simulink model "S2_Boost_model_real"  (R2021a)
settings: Solver=VariableStepAuto  StartTime=0.0  StopTime=spec.sim_time  FixedStep=1e-9  MaxStep=1e-7  RelTol=1e-3
undefined symbols (not defined in the file): real, spec
libraries: fl_lib x16, nesl_utility x12, spsMeanLib x5, ee_lib x4, spsRMSLib x3, spsPWMGeneratorDCDCLib x1
settings Model: Creator=delta  LastModifiedBy=delta
settings SolverCC: MaxConsecutiveMinStep=10  ZeroCrossAlgorithm=Adaptive
settings DebuggingCC: IgnoredZcDiagnostic=none

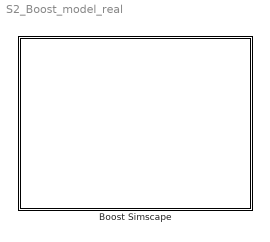
== system S2_Boost_model_real ==
  Boost Simscape : Subsystem

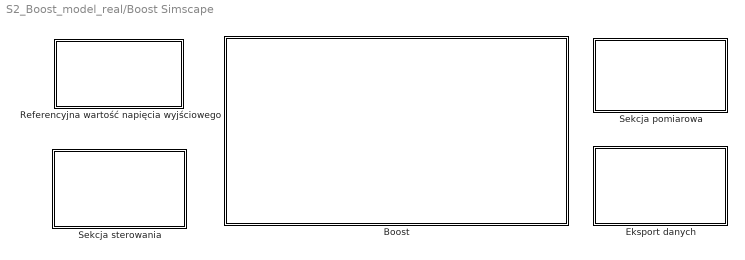
== system S2_Boost_model_real/Boost Simscape ==
  Boost : Subsystem
  Eksport danych : Subsystem
  Referencyjna wartość napięcia wyjściowego : Subsystem
  Sekcja pomiarowa : Subsystem
  Sekcja sterowania : Subsystem

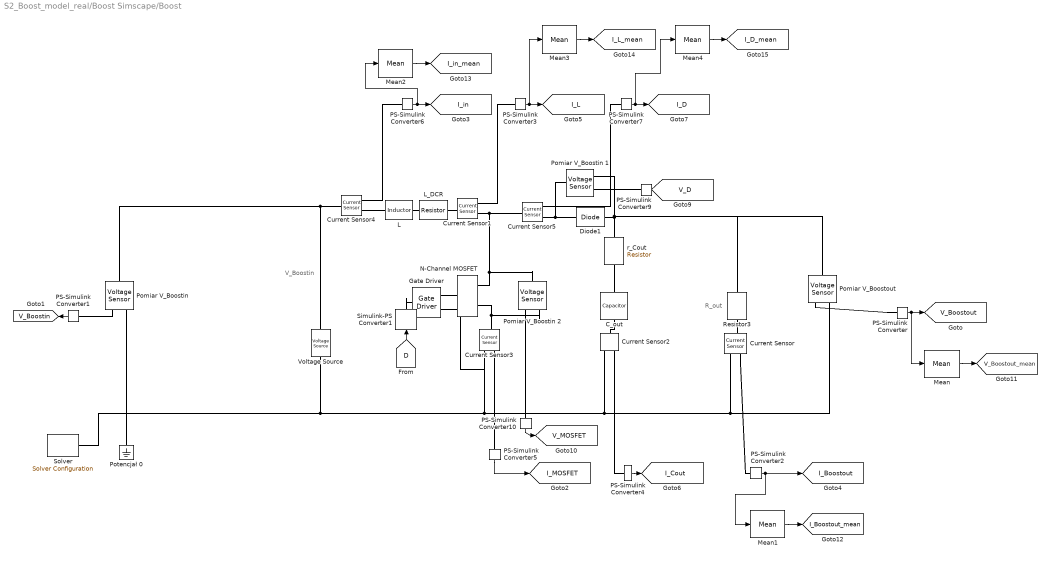
== system S2_Boost_model_real/Boost Simscape/Boost ==
  note: V_Boostin
  note: R_out
  "C_out " : fl_lib/Electrical/Electrical Elements/Capacitor  c=real.Cout.param.C_out F  r=0 Ohm  g=0 1/Ohm  i_specify=off  i_priority=None  i=0 A  i_nominal_specify=off  i_nominal_unit=A  i_nominal_value=1  v_specify=off  v_priority=None  v=0 V  v_nominal_specify=off  v_nominal_unit=V  v_nominal_value=1  vc_specify=off  vc_priority=High  vc=0 V  vc_nominal_specify=off  vc_nominal_unit=V  vc_nominal_value=1
  Current Sensor{,1..5} (6 alike) : fl_lib/Electrical/Electrical Sensors/Current Sensor
  Diode1 : ee_lib/Semiconductors & Converters/Diode  ModelType=ee.enum.diode.modelType.pwl  IfMat=[.07, .12, .19, 1.75, 4.24, 7.32, 11.2; .16, .3, .72, 2.14, 4.02, 6.35, 9.12] A  TjVec=[25, 125] degC  VfVec=[.5, .7, .9, 1.3, 1.7, 2.1, 2.5] V  Vf=real.Diode.param.V_f V  Ron=1e-9 Ohm  Goff=1e-8 S  prmExp=ee.enum.diode.expParam.useTwo  I12=[.0137, .545] A  V12=[.6, .7] V  IS=1e-12 A  ec=1  I1=0.0137 A  V1=0.6 V  RS=0 Ohm  Tmeas=25 degC  N_series=1  N_parallel=1  Rz=0.3 Ohm  BV=inf V  C_param=ee.enum.diode.capParam.fixed  CJ=5 pF  CJ0=5 pF  VJ=1 V  Mgrad=0.5  Vvec=[.1, 10, 100] V  Cvec=[3.5, 1, .4] pF  FC=0.5  Q_param=ee.enum.diode.recoveryParam.off  iRM=-7.15 A  iF=4 A  didt=-750 A/us  trr_factor=3  trr=115 ns  Qrr=150 s*nA  TT=50 ns  tau=100 ns  T_param=ee.enum.diode.temperatureParam.off  IS_T2=1.25e-7 A  I1_T2=0.245 A  V1_T2=0.5 V  Tmeas2=125 degC  EG_param=ee.enum.diode.egapParam.material_si  EG=1.11 eV  XTI_param=ee.enum.diode.xtiParam.pn  XTI=3  dBVdT=0 V/K  enable_faults=ee.enum.faults.faultEnable.no  fault_action=ee.enum.faults.faultAction.none  fault_types=ee.enum.diode.faults.open  tau_fault=1e-3 s  IfMat_faulted=[.07, .12, .19, 1.75, 4.24, 7.32, 11.2; .16, .3, .72, 2.14, 4.02, 6.35, 9.12] A  VfVec_faulted=[.5, .7, .9, 1.3, 1.7, 2.1, 2.5] V  Ropen_faulted=1000 Ohm  Gshort_faulted=1000 1/Ohm  Vf_faulted=0.6 V  Ron_faulted=0.3 Ohm  Goff_faulted=1e-8 S  I12_faulted=[.0137, .545] A  V12_faulted=[.6, .7] V  IS_faulted=1e-12 A  ec_faulted=1  I1_faulted=0.0137 A  V1_faulted=0.6 V  RS_faulted=0 Ohm  Rz_faulted=0.3 Ohm  BV_faulted=inf V  Cscale_faulted=100  enable_temporal_fault=ee.enum.faults.faultEnable.no  t_fault=inf s  enable_behavioral_fault=ee.enum.faults.faultEnable.no  max_permissible_voltage=inf V  n_fail_on_voltage=1  max_permissible_current=inf A  t_fail_on_current=1 s  max_permissible_dVdt=inf V/s  Tdevice=25 degC  i_specify=off  i_priority=None  i=0 A  i_nominal_specify=off  i_nominal_unit=A  i_nominal_value=1  v_specify=off  v_priority=None  v=0 V  v_nominal_specify=off  v_nominal_unit=V  v_nominal_value=1  i_diode_specify=off  i_diode_priority=None  i_diode=0 A  i_diode_nominal_specify=off  i_diode_nominal_unit=A  i_diode_nominal_value=1  v_diode_specify=off  v_diode_priority=None  v_diode=0 V  v_diode_nominal_specify=off  v_diode_nominal_unit=V  v_diode_nominal_value=1  i_capacitor_specify=off  i_capacitor_priority=None  i_capacitor=0 A  i_capacitor_nominal_specify=off  i_capacitor_nominal_unit=A  i_capacitor_nominal_value=1  v_capacitor_specify=off  v_capacitor_priority=None  v_capacitor=0 V  v_capacitor_nominal_specify=off  v_capacitor_nominal_unit=V  v_capacitor_nominal_value=1  power_dissipated_specify=off  power_dissipated_priority=None  power_dissipated=0 W  power_dissipated_nominal_specify=off  power_dissipated_nominal_unit=W  power_dissipated_nominal_value=1  max_permissible_temperature=inf K  t_fail_on_temperature=1 s  thermal_network_parameterization=ee.enum.thermalNetworkTopology.cauer  Rth=[0, 10] K/W  Rth_Foster=[4, 6] K/W  thermal_mass_parameterization=ee.enum.thermalNetwork.timeconstant  thermal_mass=[0, 1] J/K  thermal_mass_Foster=[1.5, 3] J/K  thermal_time_constant=[0, 10] s  thermal_time_constant_Foster=[6, 18] s  thermal_mass_initial_temperatures=[25, 25] degC
  Gate Driver : ee_lib/Semiconductors & Converters/Gate Driver  vHigh=real.MOSFET.param.V_GS V  vLow=0 V  parameterization=2  rHigh=1e-9 Ohm  rLow=1e-9 Ohm  tRise=real.MOSFET.param.t_R s  tFall=real.MOSFET.param.t_F s  cLoad=10 nF  enable_faults=0  t_fault=1 s  fault_type=1  uHighValue=0.7  uLowValue=0.3  tHigh=real.MOSFET.param.t_R s  tLow=real.MOSFET.param.t_F s  ZonTime_specify=off  ZonTime_priority=None  ZonTime=0 s  ZoffTime_specify=off  ZoffTime_priority=None  ZoffTime=0 s  uHigh=2.0 V  uLow=0.8 V
      settings: SourceProductBaseCode=PS  InternalSimscapePortConfiguration="{\"Bottom\":[],\"Left\":[{\"id\":\"u\",\"label\":\"u\",\"type\":\"input\"}],\"Right\":[{\"id\":\"G\",\"label\":\"G\",\"type\":\"foundation.electrical.electrical\"},{\"id\":\"S\",\"label\":\"S\",\"type\":\"foundation.electrical.electrical\"}],\"Top\":[]}"
  L : fl_lib/Electrical/Electrical Elements/Inductor  l=real.L.param.L H  r=0 Ohm  g=0 1/Ohm  i_specify=off  i_priority=None  i=0 A  i_nominal_specify=off  i_nominal_unit=A  i_nominal_value=1  v_specify=off  v_priority=None  v=0 V  v_nominal_specify=off  v_nominal_unit=V  v_nominal_value=1  i_L_specify=off  i_L_priority=High  i_L=0 A  i_L_nominal_specify=off  i_L_nominal_unit=A  i_L_nominal_value=1
  L_DCR : fl_lib/Electrical/Electrical Elements/Resistor  R=real.L.param.DCR Ohm  i_specify=off  i_priority=None  i=0 A  i_nominal_specify=off  i_nominal_unit=A  i_nominal_value=1  v_specify=off  v_priority=None  v=0 V  v_nominal_specify=off  v_nominal_unit=V  v_nominal_value=1
  Mean{,1..4} (5 alike) : spsMeanLib/Mean  Freq=spec.f_s  Vinit=0  Ts=0
  N-Channel MOSFET : ee_lib/Semiconductors & Converters/N-Channel MOSFET  paramTerminal=ee.enum.mosfet.numberOfTerminals.three  parameterization=ee.enum.mosfet.parameterization.datasheet  prmDatasheet=ee.enum.temperatureParameterization.none  prmEquCoeff=ee.enum.temperatureParameterization.none  Beta=5.0 A/V^2  Rds=real.MOSFET.param.R_DS Ohm  Id=real.MOSFET.param.I_D A  Vgs=real.MOSFET.param.V_GS V  Vth=real.MOSFET.param.V_th V  Vth0=1.7 V  lam=0 1/V  gamma_vth=0.5 V^0.50000  phib=0.5 V  Vth1=1.9071 V  Vbs1=-1 V  Vth2=2.066 V  Vbs2=-2 V  Tmeas=25 degC  RS=1e-9 Ohm  RD=1e-9 Ohm  RB=0.001 Ohm  C_param=ee.enum.mosfet.capacitanceParam.fixedciss  C_GS=270 pF  C_GD=80 pF  C_DS=0 pF  C_iss=real.MOSFET.param.C_iss F  C_rss=real.MOSFET.param.C_rss F  C_oss=real.MOSFET.param.C_oss F  charge_linearity_param=ee.enum.mosfet.cgdLinearity.constant  C_OX=200 pF  V_C_OX=-0.5 V  C_iss_vec=[720, 700, 590, 470, 390, 310] pF  C_rss_vec=[450, 400, 300, 190, 95, 55] pF  C_oss_vec=[900, 810, 690, 420, 270, 170] pF  C_GS_vec=[270, 300, 290, 280, 295, 255] pF  C_GD_vec=[450, 400, 300, 190, 95, 55] pF  C_DS_vec=[450, 410, 390, 230, 175, 115] pF  C_Vds_vec=[.1, .3, 1, 3, 10, 30] V  V_GS_for_cap_data=0 V  charge_linearity_param_vgb=ee.enum.mosfet.cgbLinearity.instantly  Di_param=ee.enum.mosfet.diodeParam.no  IsDiode=0 A  Vbi=0.6 V  n=1  Cj0Diode=0 pF  TT=50e-9 s  dVth_dT=-6 mV/K  dVth0_dT=-6 mV/K  Rds_T2=0.037 Ohm  Tmeas2=125 degC  BEXDatasheet=-1.5  BEXEquCoeff=-1.5  etaisDatasheet=3  etaisEquCoeff=3  Vgs_vec=[-.5, 2, 3, 4, 5] V  Vds_vec=[0, 2, 4, 8, 12, 16, 20] V  Vbs_vec=[0, -4, -6, -12] V  T_vec=[25, 125] degC  Vth_vec=[.4, 1.2, 1.4, 1.45] V  Vth_mat=[.4, .35; 1.2, 1.15; 1.4, 1.35; 1.45, 1.4] V  Ids_mat=[0, 0, 0, 0, 0, 0, 0; 0, .003, .0038, .0043, .0046, .0048, .0049; 0, .0055, .008, .009, .0095, .01, .0101; 0, .0115, .016, .018, .019, .0195, .02; 0, .0152, .0225, .0265, .028, .0295, .03] A  Ids_mat0=[0, 0, 0, 0, 0, 0, 0; 0, .003, .0038, .0043, .0046, .0048, .0049; 0, .0055, .008, .009, .0095, .01, .0101; 0, .0115, .016, .018, .019, .0195, .02; 0, .0152, .0225, .0265, .028, .0295, .03] A  Ids_mat_3D=zeros(5, 7, 2) A  Ids_mat_3D0=zeros(5, 7, 2) A  IV_table_symmetry=ee.enum.mosfet.symmetricNIV.no  VfVec=[.5, .7, .9, 1.3, 1.7, 2.1, 2.5] V  TjVec=[25, 125] degC  IfVec=[.07, .12, .19, 1.75, 4.24, 7.32, 11.2] A  IfMat=[.07, .12, .19, 1.75, 4.24, 7.32, 11.2; .16, .3, .72, 2.14, 4.02, 6.35, 9.12] A  Tmeas_dio=25 degC  etaisTabulated=3  TdeviceDatasheet=25 degC  TdeviceEquCoeff=25 degC  TdeviceTabulated=25 degC  thermal_network_parameterization=ee.enum.thermalNetworkTopology.cauer  Rth=[0, 10] K/W  Rth_Foster=[4, 6] K/W  thermal_mass_parameterization=ee.enum.thermalNetwork.timeconstant  thermal_mass=[0, 1] J/K  thermal_mass_Foster=[1.5, 3] J/K  thermal_time_constant=[0, 10] s  thermal_time_constant_Foster=[6, 18] s  thermal_mass_initial_temperatures=[25, 25] degC  betaref=18 A/V^2  Vfbref=-1.1 V  gamma=3.5 V^0.50000  phib2ref=1 V  thesatref=0.4 1/V  alpha=0  Vp=5e-2 V  thesrref=0 1/V  m=8  Tref=25 degC  Cox=1500 pF  Cgso=100 pF  Cgdo=14 pF  Rsref=2e-3 Ohm  Rdref=0.17 Ohm  Rgref=8.4 Ohm  Rbref=2e-3 Ohm  Isref=5.2e-13 A  Cj0=480 pF  Tprm=1  etabet=1.3  Stvfb=5e-4 V/K  Stphib=-8.5e-4 V/K  etasat=1.04  etasr=0.65  etar=0.95  etais=3  Tsim=25 degC  T0=[25, 25] degC
  PS-Simulink Converter{,1..7,9..10} (10 alike) : nesl_utility/PS-Simulink Converter  PhysicalDomain=network_engine_domain  SubClassName=ps_output  LeftPortType=input  RightPortType=output  PseudoPeriodic=off  Frequencies=[]  Unit=inherit  AffineConversion=off
      settings: SourceProductBaseCode=PW,SS
  "Pomiar V_Boostin " : fl_lib/Electrical/Electrical Sensors/Voltage Sensor
  Pomiar V_Boostin 1 : fl_lib/Electrical/Electrical Sensors/Voltage Sensor
  Pomiar V_Boostin 2 : fl_lib/Electrical/Electrical Sensors/Voltage Sensor
  "Pomiar V_Boostout " : fl_lib/Electrical/Electrical Sensors/Voltage Sensor
  Potencjał 0 : fl_lib/Electrical/Electrical Elements/Electrical Reference
  Resistor3 : fl_lib/Electrical/Electrical Elements/Resistor  R=real.general.calc.R_out Ohm  i_specify=off  i_priority=None  i=0 A  i_nominal_specify=off  i_nominal_unit=A  i_nominal_value=1  v_specify=off  v_priority=None  v=0 V  v_nominal_specify=off  v_nominal_unit=V  v_nominal_value=1
  Simulink-PS Converter1 : nesl_utility/Simulink-PS Converter  PhysicalDomain=network_engine_domain  SubClassName=ps_input  LeftPortType=input  RightPortType=output  PseudoPeriodic=off  Frequencies=[]  NoiseDistribution=none  NoiseParameters=[]  Unit=1  AffineConversion=off  FilteringAndDerivatives=provide  SimscapeFilterOrder=1  InputFilterTimeConstant=0.001  UdotUserProvided=0
  "Solver " : nesl_utility/Solver Configuration  PhysicalDomain=network_engine_domain  SubClassName=solver  LeftPortType=input  RightPortType=generic  Tones=[]  Harmonics=[]  SimulateNoise=off  Profile=off  UseLocalSampling=off  EnableSwitchedLinearOptims=on  FrequencyDomain=off  UseCCode=off  RelTol=0.001  AbsTol=1e-06  MinStep=1e-09  ToWorkspace=off  RevertToSquareIcSolve=off  NumHomotopyIterations=100  PhasorMode=off  PhasorModeNumHarmonics=1  DoDC=off  ResidualTolerance=1e-09  UseLocalSolver=off  LocalSolverChoice=NE_BACKWARD_EULER_ADVANCER  LocalSolverSampleTime=0.001  DoFixedCost=on  MaxNonlinIter=3  MaxModeIter=2  ComputeImpulses=off  ImpulseIterations=2  LinearAlgebra=auto  EquationFormulation=NE_TIME_EF  DelaysMemoryBudget=1024  AutomaticFiltering=on  FilteringTimeConstant=0.001  PartitionStorageMethod=AS_NEEDED  PartitionMemoryBudget=1024  PartitionMethod=ROBUST
      settings: SourceProductBaseCode=PW,SS
  Voltage Source : ee_lib/Sources/Voltage Source  dc_voltage=spec.V_in V  ac_voltage=0 V  ac_shift=0 rad  ac_frequency=60 Hz  noise_mode=0  PSD=0.2/1e3 V^2/Hz  repeatability=1  auto_seed=1019125215  user_seed=0  sample_time=1e-3 s  i_specify=off  i_priority=None  i=0 A  i_nominal_specify=off  i_nominal_unit=A  i_nominal_value=1  v_specify=off  v_priority=None  v=0 V  v_nominal_specify=off  v_nominal_unit=V  v_nominal_value=1
  r_Cout : fl_lib/Electrical/Electrical Elements/Resistor  R=real.Cout.param.ESR_Cout Ohm  i_specify=off  i_priority=None  i=0 A  i_nominal_specify=off  i_nominal_unit=A  i_nominal_value=1  v_specify=off  v_priority=None  v=0 V  v_nominal_specify=off  v_nominal_unit=V  v_nominal_value=1
  tag scope: I_Boostout=global, I_Boostout_mean=global, I_Cout=global, I_D=global, I_D_mean=global, I_L=global, I_L_mean=global, I_MOSFET=global, I_in=global, I_in_mean=global, V_Boostin=global, V_Boostout=global, V_Boostout_mean=global, V_D=global, V_MOSFET=global
  wires:
  PS-Simulink Converter/1 -> Mean/1, [V_Boostout]
  PS-Simulink Converter1/1 -> [V_Boostin]
  PS-Simulink Converter5/1 -> [I_MOSFET]
  PS-Simulink Converter9/1 -> [V_D]
  PS-Simulink Converter10/1 -> [V_MOSFET]
  PS-Simulink Converter4/1 -> [I_Cout]
  [D] -> Simulink-PS Converter1/1
  Mean/1 -> [V_Boostout_mean]
  PS-Simulink Converter2/1 -> Mean1/1, [I_Boostout]
  Mean1/1 -> [I_Boostout_mean]
  PS-Simulink Converter6/1 -> Mean2/1, [I_in]
  Mean2/1 -> [I_in_mean]
  PS-Simulink Converter3/1 -> Mean3/1, [I_L]
  Mean3/1 -> [I_L_mean]
  PS-Simulink Converter7/1 -> Mean4/1, [I_D]
  Mean4/1 -> [I_D_mean]
  connections:
  Current Sensor/LConn1 -- Resistor3/RConn1
  Current Sensor1/RConn2 -- N-Channel MOSFET/RConn1 -- Pomiar V_Boostin 2/LConn1 -- Current Sensor5/LConn1
  "C_out "/RConn1 -- Current Sensor2/LConn1
  PS-Simulink Converter4/LConn1 -- Current Sensor2/RConn1
  Current Sensor/RConn2 -- Voltage Source/RConn1 -- "Solver "/RConn1 -- Potencjał 0/LConn1 -- "Pomiar V_Boostin "/RConn2 -- Gate Driver/RConn2 -- Current Sensor3/RConn2 -- Current Sensor2/RConn2 -- "Pomiar V_Boostout "/RConn2
  "C_out "/LConn1 -- r_Cout/RConn1
  Current Sensor/RConn1 -- PS-Simulink Converter2/LConn1
  PS-Simulink Converter3/LConn1 -- Current Sensor1/RConn1
  PS-Simulink Converter/LConn1 -- "Pomiar V_Boostout "/RConn1
  PS-Simulink Converter1/LConn1 -- "Pomiar V_Boostin "/RConn1
  Current Sensor3/LConn1 -- N-Channel MOSFET/RConn2 -- Pomiar V_Boostin 2/RConn2
  PS-Simulink Converter5/LConn1 -- Current Sensor3/RConn1
  Current Sensor4/RConn2 -- L/LConn1
  Current Sensor4/RConn1 -- PS-Simulink Converter6/LConn1
  Current Sensor5/RConn2 -- Diode1/LConn1 -- Pomiar V_Boostin 1/LConn1
  Current Sensor5/RConn1 -- PS-Simulink Converter7/LConn1
  PS-Simulink Converter9/LConn1 -- Pomiar V_Boostin 1/RConn1
  PS-Simulink Converter10/LConn1 -- Pomiar V_Boostin 2/RConn1
  Pomiar V_Boostin 1/RConn2 -- Diode1/RConn1 -- r_Cout/LConn1 -- "Pomiar V_Boostout "/LConn1 -- Resistor3/LConn1
  L_DCR/LConn1 -- L/RConn1
  L_DCR/RConn1 -- Current Sensor1/LConn1
  "Pomiar V_Boostin "/LConn1 -- Voltage Source/LConn1 -- Current Sensor4/LConn1
  Simulink-PS Converter1/RConn1 -- Gate Driver/LConn1
  Gate Driver/RConn1 -- N-Channel MOSFET/LConn1

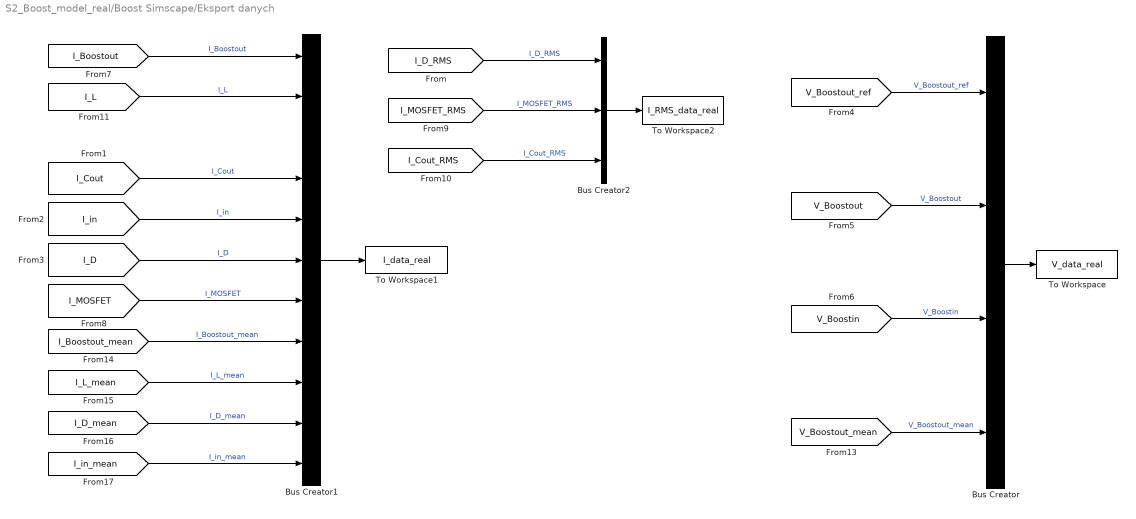
== system S2_Boost_model_real/Boost Simscape/Eksport danych ==
  Bus Creator : BusCreator  Inputs=4
  Bus Creator1 : BusCreator  Inputs=11
  Bus Creator2 : BusCreator  Inputs=3
  To Workspace : ToWorkspace  VariableName=V_data_real  SaveFormat=Timeseries  SampleTime=-1
  To Workspace1 : ToWorkspace  VariableName=I_data_real  SaveFormat=Timeseries  SampleTime=-1
  To Workspace2 : ToWorkspace  VariableName=I_RMS_data_real  SaveFormat=Timeseries  SampleTime=-1
  wires:
  [V_Boostin] -> Bus Creator/3  "V_Boostin"
  Bus Creator/1 -> To Workspace/1
  [V_Boostout_ref] -> Bus Creator/1  "V_Boostout_ref"
  [V_Boostout] -> Bus Creator/2  "V_Boostout"
  [I_Boostout] -> Bus Creator1/1  "I_Boostout"
  [I_Cout] -> Bus Creator1/4  "I_Cout"
  [I_L] -> Bus Creator1/2  "I_L"
  [I_in] -> Bus Creator1/5  "I_in"
  [I_D] -> Bus Creator1/6  "I_D"
  [I_MOSFET] -> Bus Creator1/7  "I_MOSFET"
  Bus Creator1/1 -> To Workspace1/1
  [I_D_RMS] -> Bus Creator2/1  "I_D_RMS"
  [I_MOSFET_RMS] -> Bus Creator2/2  "I_MOSFET_RMS"
  Bus Creator2/1 -> To Workspace2/1
  [I_Cout_RMS] -> Bus Creator2/3  "I_Cout_RMS"
  [V_Boostout_mean] -> Bus Creator/4  "V_Boostout_mean"
  [I_Boostout_mean] -> Bus Creator1/8  "I_Boostout_mean"
  [I_L_mean] -> Bus Creator1/9  "I_L_mean"
  [I_D_mean] -> Bus Creator1/10  "I_D_mean"
  [I_in_mean] -> Bus Creator1/11  "I_in_mean"

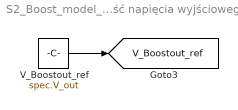
== system S2_Boost_model_real/Boost Simscape/Referencyjna wartość napięcia wyjściowego ==
  V_Boostout_ref : Constant  Value=spec.V_out
  tag scope: V_Boostout_ref=global
  wires:
  V_Boostout_ref/1 -> [V_Boostout_ref]

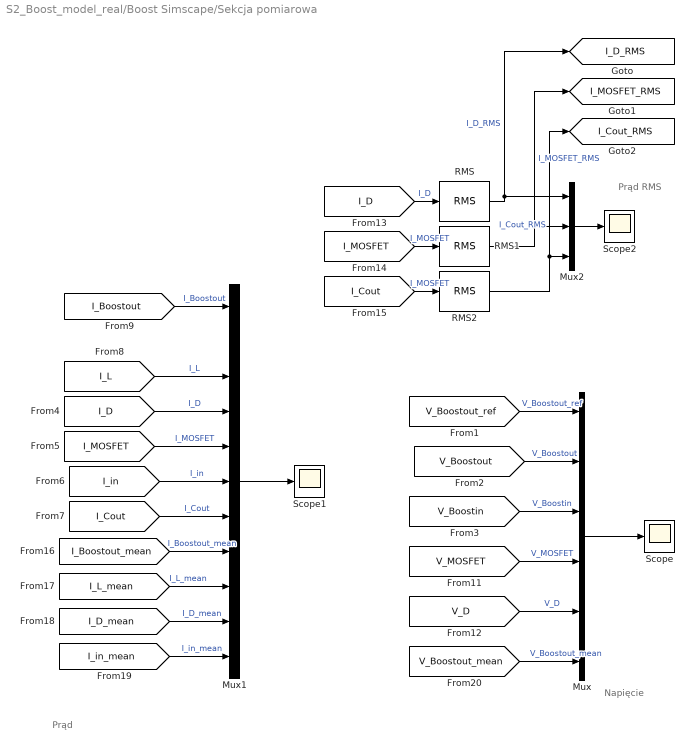
== system S2_Boost_model_real/Boost Simscape/Sekcja pomiarowa ==
  note: Napięcie
  note: Prąd
  note: Prąd RMS
  Mux : Mux  Inputs=6
  Mux1 : Mux  Inputs=11
  Mux2 : Mux  Inputs=3
  RMS : spsRMSLib/RMS  TrueRMS=on  Freq=spec.f_s  RMSInit=0  Ts=0
  RMS1 : spsRMSLib/RMS  TrueRMS=on  Freq=spec.f_s  RMSInit=0  Ts=0
  RMS2 : spsRMSLib/RMS  TrueRMS=on  Freq=spec.f_s  RMSInit=0  Ts=0
  Scope : Scope
  Scope1 : Scope
  Scope2 : Scope
  tag scope: I_Cout_RMS=global, I_D_RMS=global, I_MOSFET_RMS=global
  wires:
  [V_Boostout_ref] -> Mux/1  "V_Boostout_ref"
  [I_L] -> Mux1/3  "I_L"
  Mux/1 -> Scope/1
  Mux1/1 -> Scope1/1
  [V_Boostin] -> Mux/3  "V_Boostin"
  [I_Boostout] -> Mux1/1  "I_Boostout"
  [V_Boostout] -> Mux/2  "V_Boostout"
  [I_MOSFET] -> Mux1/5  "I_MOSFET"
  [I_D] -> Mux1/4  "I_D"
  [I_in] -> Mux1/6  "I_in"
  [I_Cout] -> Mux1/7  "I_Cout"
  [V_MOSFET] -> Mux/4  "V_MOSFET"
  [V_D] -> Mux/5  "V_D"
  [I_D] -> RMS/1  "I_D"
  [I_MOSFET] -> RMS1/1  "I_MOSFET"
  RMS/1 -> [I_D_RMS], Mux2/1  "I_D_RMS"
  RMS1/1 -> [I_MOSFET_RMS], Mux2/2  "I_MOSFET_RMS"
  Mux2/1 -> Scope2/1
  [I_Cout] -> RMS2/1  "I_MOSFET"
  RMS2/1 -> Mux2/3, [I_Cout_RMS]  "I_Cout_RMS"
  [I_in_mean] -> Mux1/11  "I_in_mean"
  [I_Boostout_mean] -> Mux1/8  "I_Boostout_mean"
  [I_D_mean] -> Mux1/10  "I_D_mean"
  [I_L_mean] -> Mux1/9  "I_L_mean"
  [V_Boostout_mean] -> Mux/6  "V_Boostout_mean"

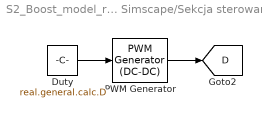
== system S2_Boost_model_real/Boost Simscape/Sekcja sterowania ==
  Duty : Constant  Value=real.general.calc.D
  "PWM Generator " : spsPWMGeneratorDCDCLib/PWM Generator (DC-DC)  Fsw=spec.f_s  Ts=0
  tag scope: D=global
  wires:
  "PWM Generator "/1 -> [D]
  Duty/1 -> "PWM Generator "/1
